simulink model "PID"  (R2023a)
settings: Solver=FixedStepAuto  StartTime=0.0  StopTime=inf  FixedStep=.01  RelTol=1e-3
undefined symbols (not defined in the file or in its folder): angular, linear
libraries: ros2lib x16

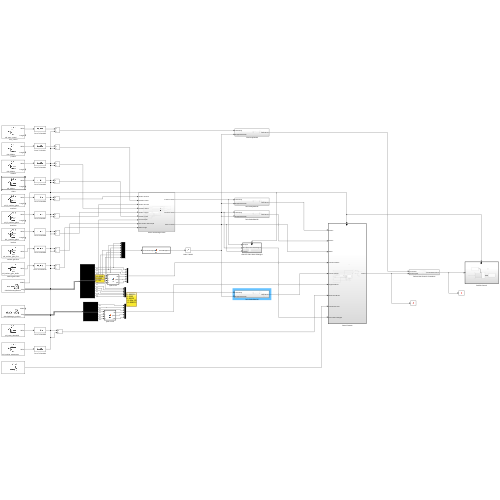
[thumbnail: Simulink's stored preview of the top-level diagram]
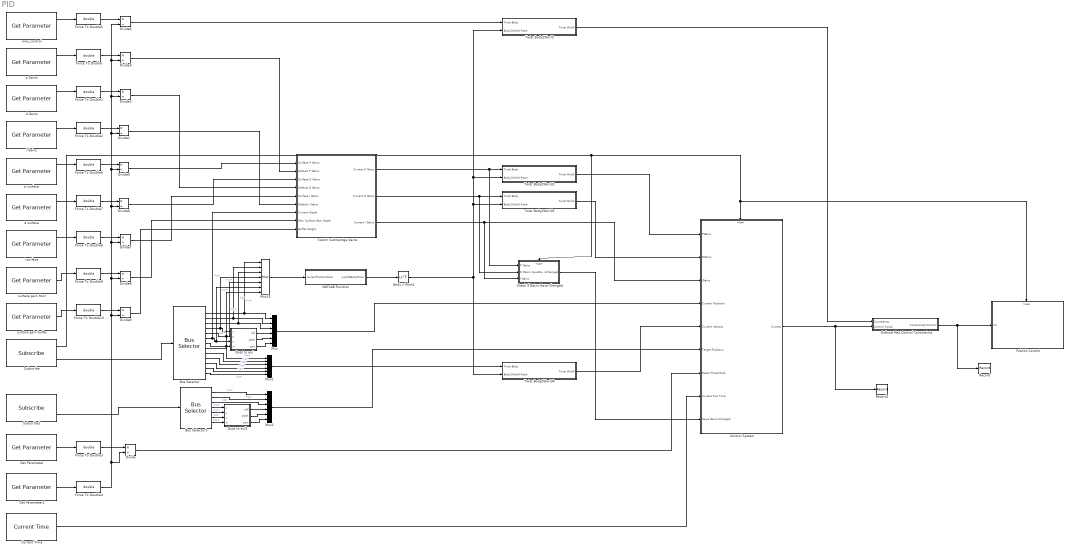
== system PID ==
  Body 2 World : Math  Operator=transpose
  Bus Selector : BusSelector  OutputSignals=pose.pose.position.x,pose.pose.position.y,pose.pose.position.z,pose.pose.orientation.x,pose.pose.orientation.y,pose.pose.orientation.z,pose.pose.orientation.w,twist.twist.linear.x,twist.twist.linear.y,twist.twist.linear.z,twist.twist.angular.x,twist.twist.angular.y,twist.twist.angular.z
  Bus Selector1 : BusSelector  OutputSignals=position.x,position.y,position.z,orientation.x,orientation.y,orientation.z,orientation.w
  Check if Gains Have Changed : Subsystem
  Control System : Subsystem
  Current Time : ros2lib/Current Time  OutputFormat=double  SampleTime=-1  ModelName=PID
  Divide{,1..9} (10 alike) : Product  Inputs=*/
  Enforce Max Control Constraints : Subsystem
  Force To Double{,1..10} (11 alike) : DataTypeConversion  OutDataTypeStr=double  SaturateOnIntegerOverflow=off  RndMeth=Floor
  Get Parameter : ros2lib/Get Parameter  ParameterName=pid_reset_threshold  ParameterType=int64  ParameterMaxArrayLength=16  ParameterInitialValue=100000  SampleTime=-1  ModelName=PID  BlockId=ParamGet_PID_43
  Get Parameter1 : ros2lib/Get Parameter  ParameterName=pid_scaling_parameters  ParameterType=int64  ParameterMaxArrayLength=16  ParameterInitialValue=1000000  SampleTime=-1  ModelName=PID  BlockId=ParamGet_PID_44
  MATLAB Function : MATLAB Function  TreatAsAtomicUnit=on
  Mux : Mux  Inputs=6
  Mux1 : Mux  Inputs=6
  Mux15 : Mux  Inputs=7
  Mux2 : Mux  Inputs=6
  Publish Control : Subsystem
  Quat to eul : MATLAB Function  TreatAsAtomicUnit=on
  Quat to eul1 : MATLAB Function  TreatAsAtomicUnit=on
  Record : Record  FileSettingsInternal="{\"entries\":[{\"content\":{\"excelSettings\":{\"content\":{},\"type\":\"Streamout.ExcelSettings\"}},\"type\":\"Streamout.FileSettingStorage\",\"uuid\":\"\"}],\"packageUris\":[\"http:\\/\\/schema.mathworks.com\\/mf0\\/streamout_blocks\\/R2020a\"],\"version\":\"1.0\"}"  Layout=[1 1]  SignalsInternal="{\"entries\":[{\"content\":{\"signals\":[{\"content\":{\"blockPath\":[],\"dimensions\":[1,6],\"domain\":\"\",\"hasChildren\":true,\"lineColor\":\"#0072bd\",\"port\":1,\"sid\":[\"\"],\"signalID\":55033,\"signalName\":\"Enforce Max Control Constraints\"},\"type\":\"RecordBlkView.Signal\",\"uuid\":\"\"},{\"content\":{\"blockPath\":[],\"channel\":[1,1],\"dimensions\":[1,6],\"domain\":\"\",\"lineColor\":\"#d95319\",\"parentID\":55033,\"port\":1,\"sid\":[\"\"],\"signal ...(+1475 chars)"  VisualizationBindings="{\"sparklinesplugin\":{\"info\":[{\"bindingParametersList\":[],\"subplotID\":1}]}}"
  Record1 : Record  FileSettingsInternal="{\"entries\":[{\"content\":{\"excelSettings\":{\"content\":{},\"type\":\"Streamout.ExcelSettings\"}},\"type\":\"Streamout.FileSettingStorage\",\"uuid\":\"\"}],\"packageUris\":[\"http:\\/\\/schema.mathworks.com\\/mf0\\/streamout_blocks\\/R2020a\"],\"version\":\"1.0\"}"  Layout=[1 1]  SignalsInternal="{\"entries\":[{\"content\":{\"signals\":[{\"content\":{\"blockPath\":[],\"dimensions\":[1,6],\"domain\":\"\",\"hasChildren\":true,\"lineColor\":\"#edb120\",\"port\":1,\"sid\":[\"\"],\"signalID\":55038,\"signalName\":\"Control System\"},\"type\":\"RecordBlkView.Signal\",\"uuid\":\"\"},{\"content\":{\"blockPath\":[],\"channel\":[1,1],\"dimensions\":[1,6],\"domain\":\"\",\"lineColor\":\"#64d413\",\"parentID\":55038,\"plots\":[1],\"port\":1,\"sid\":[\"\"],\"signalID\":5 ...(+1356 chars)"  VisualizationBindings="{\"sparklinesplugin\":{\"info\":[{\"bindingParametersList\":[],\"subplotID\":1}]}}"
  Subscribe : ros2lib/Subscribe  topicSource=Specify your own  topic=/talos/odometry/filtered  messageType=nav_msgs/Odometry  sampleTime=-1  QOSHistory=Keep last  QOSDepth=1  QOSReliability=Reliable  QOSDurability=Volatile
  Subscribe1 : ros2lib/Subscribe  topicSource=Specify your own  topic=/talos/pid/target_position  messageType=geometry_msgs/Pose  sampleTime=-1  QOSHistory=Keep last  QOSDepth=1  QOSReliability=Reliable  QOSDurability=Volatile
  Switch Submerdge Gains : Subsystem
  Twist Body2World : Subsystem
  Twist Body2World1 : Subsystem
  Twist Body2World2 : Subsystem
  Twist Body2World4 : Subsystem
  d Gains : ros2lib/Get Parameter  ParameterName=pid_DGains  ParameterType=int64[]  ParameterMaxArrayLength=6  ParameterInitialValue=[0,0,0,0,0,0]  SampleTime=-1  ModelName=PID  BlockId=ParamGet_PID_47
  d surface : ros2lib/Get Parameter  ParameterName=pid_D_surface_gains  ParameterType=int64[]  ParameterMaxArrayLength=6  ParameterInitialValue=[0,0,0,0,0,0]  SampleTime=-1  ModelName=PID  BlockId=ParamGet_PID_233
  i Gains : ros2lib/Get Parameter  ParameterName=pid_IGains  ParameterType=int64[]  ParameterMaxArrayLength=6  ParameterInitialValue=[0,0,0,0,0,0]  SampleTime=-1  ModelName=PID  BlockId=ParamGet_PID_46
  i surface : ros2lib/Get Parameter  ParameterName=pid_I_surface_gains  ParameterType=int64[]  ParameterMaxArrayLength=6  ParameterInitialValue=[0,0,0,0,0,0]  SampleTime=-1  ModelName=PID  BlockId=ParamGet_PID_234
  max_control : ros2lib/Get Parameter  ParameterName=pid_max_control  ParameterType=int64[]  ParameterMaxArrayLength=6  ParameterInitialValue=[0,0,0,0,0,0]  SampleTime=-1  ModelName=PID  BlockId=ParamGet_PID_123
  p Gains : ros2lib/Get Parameter  ParameterName=pid_PGains  ParameterType=int64[]  ParameterMaxArrayLength=6  ParameterInitialValue=[0,0,0,0,0,0]  SampleTime=-1  ModelName=PID  BlockId=ParamGet_PID_48
  p surface : ros2lib/Get Parameter  ParameterName=pid_P_surface_gains  ParameterType=int64[]  ParameterMaxArrayLength=6  ParameterInitialValue=[0,0,0,0,0,0]  SampleTime=-1  ModelName=PID  BlockId=ParamGet_PID_235
  surface gain buffer : ros2lib/Get Parameter  ParameterName=pid_surface_gain_buffer  ParameterType=int64  ParameterMaxArrayLength=6  ParameterInitialValue=250000  SampleTime=-1  ModelName=PID  BlockId=ParamGet_PID_239
  surface gain floor : ros2lib/Get Parameter  ParameterName=pid_surface_gain_floor  ParameterType=int64  ParameterMaxArrayLength=6  ParameterInitialValue=-750000  SampleTime=-1  ModelName=PID  BlockId=ParamGet_PID_240
  wires:
  Subscribe/2 -> Bus Selector/1
  Bus Selector/4 -> Mux15/4, Quat to eul/1(x)  "<x>"
  Bus Selector/5 -> Mux15/5, Quat to eul/2(y)  "<y>"
  Bus Selector/6 -> Switch Submerdge Gains/7(Current Depth), Mux15/6, Quat to eul/3(z)  "<z>"
  Bus Selector/7 -> Mux15/7, Quat to eul/4(w)  "<w>"
  Quat to eul/3(yaw) -> Mux/6
  Quat to eul/2(pitch) -> Mux/5
  Quat to eul/1(roll) -> Mux/4
  Bus Selector/1 -> Mux15/1, Mux/1  "<x>"
  Bus Selector/2 -> Mux15/2, Mux/2  "<y>"
  Bus Selector/3 -> Mux15/3, Mux/3  "<z>"
  Bus Selector/9 -> Mux1/2  "<y>"
  Bus Selector/8 -> Mux1/1  "<x>"
  Bus Selector/10 -> Mux1/3  "<z>"
  Bus Selector/11 -> Mux1/4  "<x>"
  Bus Selector/12 -> Mux1/5  "<y>"
  Bus Selector/13 -> Mux1/6  "<z>"
  Mux/1 -> Control System/4(Current Positions)
  Subscribe1/2 -> Bus Selector1/1
  Quat to eul1/1(roll) -> Mux2/4
  Quat to eul1/3(yaw) -> Mux2/6
  Quat to eul1/2(pitch) -> Mux2/5
  Get Parameter/1 -> Force To Double3/1
  Get Parameter1/1 -> Force To Double4/1
  Divide/1 -> Control System/7(Reset Threshhold)
  i Gains/1 -> Force To Double2/1
  d Gains/1 -> Force To Double1/1
  p Gains/1 -> Force To Double/1
  Force To Double3/1 -> Divide/1
  Mux2/1 -> Control System/6(Target Positions)
  Bus Selector1/1 -> Mux2/1  "<x>"
  Bus Selector1/2 -> Mux2/2  "<y>"
  Bus Selector1/4 -> Quat to eul1/1(x)  "<x>"
  Bus Selector1/5 -> Quat to eul1/2(y)  "<y>"
  Bus Selector1/6 -> Quat to eul1/3(z)  "<z>"
  Bus Selector1/7 -> Quat to eul1/4(w)  "<w>"
  Bus Selector1/3 -> Mux2/3  "<z>"
  Force To Double2/1 -> Divide1/1
  Force To Double1/1 -> Divide2/1
  Force To Double/1 -> Divide3/1
  Subscribe/1 -> Check if Gains Have Changed/Trigger, Publish Control/Trigger, Control System/Trigger
  MATLAB Function/1(world2BodyRotm) -> Body 2 World/1
  Twist Body2World4/1(Twist World) -> Control System/5(Current Velocity)
  Body 2 World/1 -> Twist Body2World4/2(Body2World Rotm), Twist Body2World2/2(Body2World Rotm), Twist Body2World/2(Body2World Rotm), Twist Body2World1/2(Body2World Rotm)
  Mux15/1 -> MATLAB Function/1(currentPositionQuat)
  max_control/1 -> Force To Double5/1
  Force To Double5/1 -> Divide4/1
  Divide4/1 -> Twist Body2World/1(Twist Body)
  Switch Submerdge Gains/3(Current I Gains) -> Check if Gains Have Changed/3(I Gains), Control System/3(IGains)
  Twist Body2World2/1(Twist World) -> Control System/2(DGains)
  Twist Body2World1/1(Twist World) -> Control System/1(PGains)
  Mux1/1 -> Twist Body2World4/1(Twist Body)
  Twist Body2World/1(Twist World) -> Enforce Max Control Constraints/1(Constraints)
  Control System/1(Control) -> Record1/1, Enforce Max Control Constraints/2(Control Inputs)
  Enforce Max Control Constraints/1(Constrained Control) -> Record/1, Publish Control/1(In1)
  Divide3/1 -> Switch Submerdge Gains/2(Default P Gains)
  Divide2/1 -> Switch Submerdge Gains/4(Default D Gains)
  Divide1/1 -> Switch Submerdge Gains/6(Default I Gains)
  d surface/1 -> Force To Double7/1
  p surface/1 -> Force To Double6/1
  i surface/1 -> Force To Double8/1
  Force To Double8/1 -> Divide7/1
  Force To Double7/1 -> Divide6/1
  Force To Double6/1 -> Divide5/1
  Divide5/1 -> Switch Submerdge Gains/1(Surface P Gains)
  Divide6/1 -> Switch Submerdge Gains/3(Surface D Gains)
  Divide7/1 -> Switch Submerdge Gains/5(Surface I Gains)
  surface gain floor/1 -> Force To Double9/1
  surface gain buffer/1 -> Force To Double10/1
  Force To Double10/1 -> Divide9/1
  Force To Double9/1 -> Divide8/1
  Divide8/1 -> Switch Submerdge Gains/8(Max Surface Gain Depth)
  Divide9/1 -> Switch Submerdge Gains/9(Buffer Height)
  Force To Double4/1 -> Divide/2, Divide9/2, Divide8/2, Divide7/2, Divide6/2, Divide5/2, Divide2/2, Divide3/2, Divide4/2, Divide1/2
  Current Time/1 -> Control System/8(Current Ros Time)
  Switch Submerdge Gains/1(Current P Gains) -> Check if Gains Have Changed/1(P Gains), Twist Body2World1/1(Twist Body)
  Switch Submerdge Gains/2(Current D Gains) -> Check if Gains Have Changed/2(D Gains), Twist Body2World2/1(Twist Body)
  Check if Gains Have Changed/1(haveGainsChanged) -> Control System/9(Have Gains Changed)

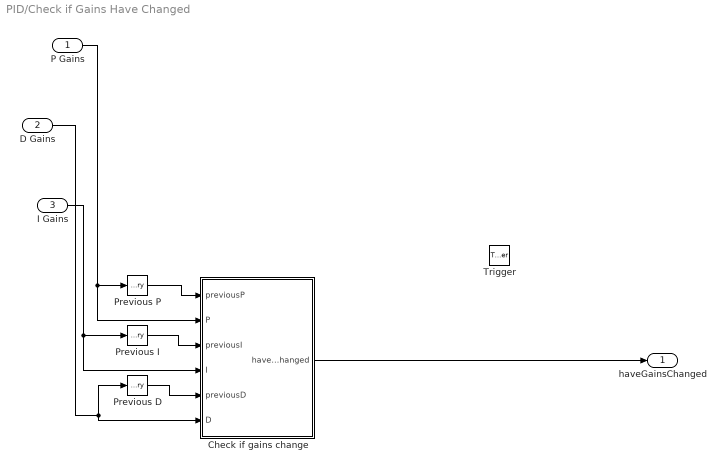
== system PID/Check if Gains Have Changed ==
  P Gains : Inport
  D Gains : Inport  Port=2
  I Gains : Inport  Port=3
  Trigger : TriggerPort  VariantControl=(inherit)  PortDimensions=1
  Check if gains change : MATLAB Function  TreatAsAtomicUnit=on
  Previous D : Memory  InheritSampleTime=on
  Previous I : Memory  InheritSampleTime=on
  Previous P : Memory  InheritSampleTime=on
  haveGainsChanged : Outport
  wires:
  I Gains/1 -> Check if gains change/4(I), Previous I/1
  Previous I/1 -> Check if gains change/3(previousI)
  Previous P/1 -> Check if gains change/1(previousP)
  P Gains/1 -> Check if gains change/2(P), Previous P/1
  Previous D/1 -> Check if gains change/5(previousD)
  D Gains/1 -> Previous D/1, Check if gains change/6(D)
  Check if gains change/1(haveGainsChanged) -> haveGainsChanged/1

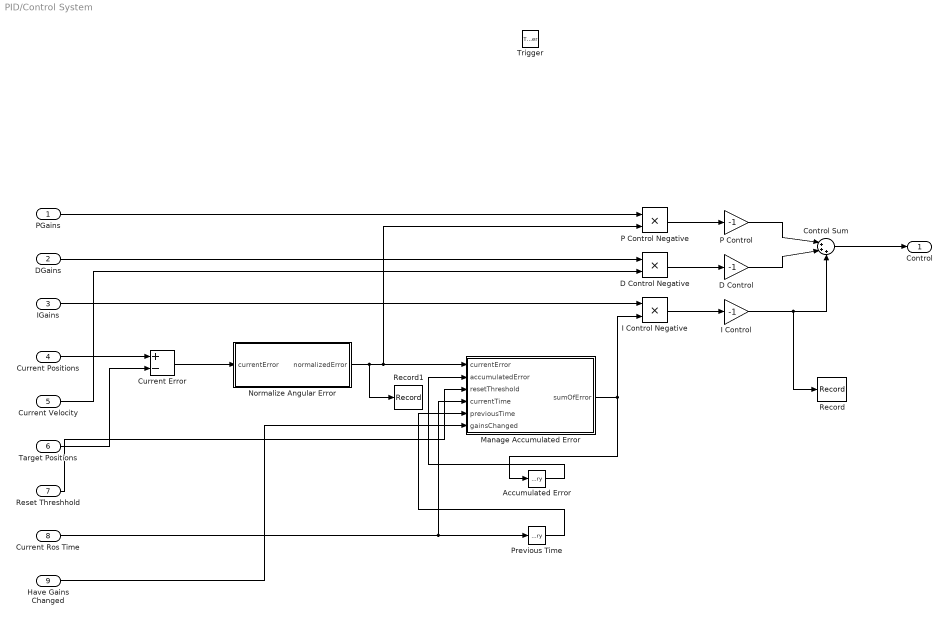
== system PID/Control System ==
  PGains : Inport
  DGains : Inport  Port=2
  IGains : Inport  Port=3
  Current Positions : Inport  Port=4
  Current Velocity : Inport  Port=5
  Target Positions : Inport  Port=6
  Reset Threshhold : Inport  Port=7
  Current Ros Time : Inport  Port=8
  Have Gains Changed : Inport  Port=9
  Trigger : TriggerPort  VariantControl=(inherit)  PortDimensions=1
  Accumulated Error : Memory  InheritSampleTime=on
  Control Sum : Sum  Inputs=|+++
  Current Error : Sum  Inputs=+-
  D Control : Gain  Gain=-1
  D Control Negative : Product
  I Control : Gain  Gain=-1
  I Control Negative : Product
  Manage Accumulated Error : MATLAB Function  TreatAsAtomicUnit=on
  Normalize Angular Error : MATLAB Function  TreatAsAtomicUnit=on
  P Control : Gain  Gain=-1
  P Control Negative : Product
  Previous Time : Memory  InitialCondition=-1  InheritSampleTime=on
  Record : Record  FileSettingsInternal="{\"entries\":[{\"content\":{\"excelSettings\":{\"content\":{},\"type\":\"Streamout.ExcelSettings\"}},\"type\":\"Streamout.FileSettingStorage\",\"uuid\":\"\"}],\"packageUris\":[\"http:\\/\\/schema.mathworks.com\\/mf0\\/streamout_blocks\\/R2020a\"],\"version\":\"1.0\"}"  Layout=[1 1]  SignalsInternal="{\"entries\":[{\"content\":{\"signals\":[{\"content\":{\"blockPath\":[],\"dimensions\":[1,6],\"domain\":\"\",\"hasChildren\":true,\"lineColor\":\"#64d413\",\"port\":1,\"sid\":[\"\"],\"signalID\":55023,\"signalName\":\"I Control\"},\"type\":\"RecordBlkView.Signal\",\"uuid\":\"\"},{\"content\":{\"blockPath\":[],\"channel\":[1,1],\"dimensions\":[1,6],\"domain\":\"\",\"lineColor\":\"#7e2f8e\",\"parentID\":55023,\"port\":1,\"sid\":[\"\"],\"signalID\":55024,\"signalName\" ...(+1297 chars)"  VisualizationBindings="{\"sparklinesplugin\":{\"info\":[{\"bindingParametersList\":[],\"subplotID\":1}]}}"
  Record1 : Record  FileSettingsInternal="{\"entries\":[{\"content\":{\"excelSettings\":{\"content\":{},\"type\":\"Streamout.ExcelSettings\"}},\"type\":\"Streamout.FileSettingStorage\",\"uuid\":\"\"}],\"packageUris\":[\"http:\\/\\/schema.mathworks.com\\/mf0\\/streamout_blocks\\/R2020a\"],\"version\":\"1.0\"}"  Layout=[1 1]  SignalsInternal="{\"entries\":[{\"content\":{\"signals\":[{\"content\":{\"blockPath\":[],\"dimensions\":[1,6],\"domain\":\"\",\"hasChildren\":true,\"lineColor\":\"#fe330a\",\"port\":1,\"sid\":[\"\"],\"signalID\":55028,\"signalName\":\"Normalize Angular Error\"},\"type\":\"RecordBlkView.Signal\",\"uuid\":\"\"},{\"content\":{\"blockPath\":[],\"channel\":[1,1],\"dimensions\":[1,6],\"domain\":\"\",\"lineColor\":\"#edb120\",\"parentID\":55028,\"port\":1,\"sid\":[\"\"],\"signalID\":5502 ...(+1419 chars)"  VisualizationBindings="{\"sparklinesplugin\":{\"info\":[{\"bindingParametersList\":[],\"subplotID\":1}]}}"
  Control : Outport
  wires:
  Reset Threshhold/1 -> Manage Accumulated Error/3(resetThreshold)
  Current Positions/1 -> Current Error/1
  I Control/1 -> Record/1, Control Sum/3
  Current Velocity/1 -> D Control Negative/2
  P Control/1 -> Control Sum/1
  D Control Negative/1 -> D Control/1
  P Control Negative/1 -> P Control/1
  Accumulated Error/1 -> Manage Accumulated Error/2(accumulatedError)
  D Control/1 -> Control Sum/2
  Manage Accumulated Error/1(sumOfError) -> I Control Negative/2, Accumulated Error/1
  I Control Negative/1 -> I Control/1
  Control Sum/1 -> Control/1
  Target Positions/1 -> Current Error/2
  Current Error/1 -> Normalize Angular Error/1(currentError)
  Normalize Angular Error/1(normalizedError) -> Record1/1, P Control Negative/2, Manage Accumulated Error/1(currentError)
  Previous Time/1 -> Manage Accumulated Error/5(previousTime)
  Current Ros Time/1 -> Manage Accumulated Error/4(currentTime), Previous Time/1
  IGains/1 -> I Control Negative/1
  PGains/1 -> P Control Negative/1
  DGains/1 -> D Control Negative/1
  Have Gains Changed/1 -> Manage Accumulated Error/6(gainsChanged)

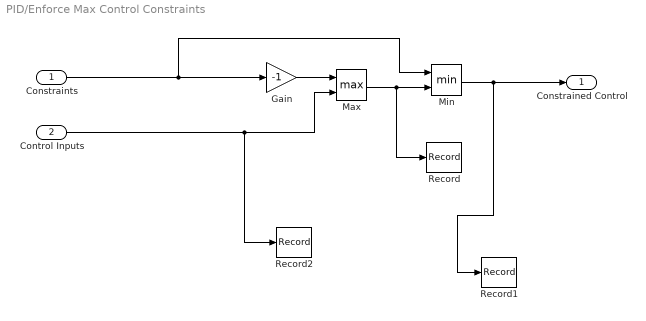
== system PID/Enforce Max Control Constraints ==
  Constraints : Inport
  Control Inputs : Inport  Port=2
  Gain : Gain  Gain=-1
  Max : MinMax  Function=max  Inputs=2
  Min : MinMax  Inputs=2
  Record : Record  FileSettingsInternal="{\"entries\":[{\"content\":{\"excelSettings\":{\"content\":{},\"type\":\"Streamout.ExcelSettings\"}},\"type\":\"Streamout.FileSettingStorage\",\"uuid\":\"\"}],\"packageUris\":[\"http:\\/\\/schema.mathworks.com\\/mf0\\/streamout_blocks\\/R2020a\"],\"version\":\"1.0\"}"  Layout=[1 1]  SignalsInternal="{\"entries\":[{\"content\":{\"signals\":[{\"content\":{\"blockPath\":[],\"dimensions\":[1,6],\"domain\":\"\",\"hasChildren\":true,\"lineColor\":\"#77ac30\",\"port\":1,\"sid\":[\"\"],\"signalID\":55043,\"signalName\":\"Max\"},\"type\":\"RecordBlkView.Signal\",\"uuid\":\"\"},{\"content\":{\"blockPath\":[],\"channel\":[1,1],\"dimensions\":[1,6],\"domain\":\"\",\"lineColor\":\"#0072bd\",\"parentID\":55043,\"port\":1,\"sid\":[\"\"],\"signalID\":55044,\"signalName\":\"Max\" ...(+1255 chars)"  VisualizationBindings="{\"sparklinesplugin\":{\"info\":[{\"bindingParametersList\":[],\"subplotID\":1}]}}"
  Record1 : Record  FileSettingsInternal="{\"entries\":[{\"content\":{\"excelSettings\":{\"content\":{},\"type\":\"Streamout.ExcelSettings\"}},\"type\":\"Streamout.FileSettingStorage\",\"uuid\":\"\"}],\"packageUris\":[\"http:\\/\\/schema.mathworks.com\\/mf0\\/streamout_blocks\\/R2020a\"],\"version\":\"1.0\"}"  Layout=[1 1]  SignalsInternal="{\"entries\":[{\"content\":{\"signals\":[{\"content\":{\"blockPath\":[],\"dimensions\":[1,6],\"domain\":\"\",\"hasChildren\":true,\"lineColor\":\"#a2142f\",\"port\":1,\"sid\":[\"\"],\"signalID\":55048,\"signalName\":\"Min\"},\"type\":\"RecordBlkView.Signal\",\"uuid\":\"\"},{\"content\":{\"blockPath\":[],\"channel\":[1,1],\"dimensions\":[1,6],\"domain\":\"\",\"lineColor\":\"#b746ff\",\"parentID\":55048,\"port\":1,\"sid\":[\"\"],\"signalID\":55049,\"signalName\":\"Min\" ...(+188 chars)"  VisualizationBindings="{\"sparklinesplugin\":{\"info\":[{\"bindingParametersList\":[],\"subplotID\":1}]}}"
  Record2 : Record  FileSettingsInternal="{\"entries\":[{\"content\":{\"excelSettings\":{\"content\":{},\"type\":\"Streamout.ExcelSettings\"}},\"type\":\"Streamout.FileSettingStorage\",\"uuid\":\"\"}],\"packageUris\":[\"http:\\/\\/schema.mathworks.com\\/mf0\\/streamout_blocks\\/R2020a\"],\"version\":\"1.0\"}"  Layout=[1 1]  SignalsInternal="{\"entries\":[{\"content\":{\"signals\":[{\"content\":{\"blockPath\":[],\"dimensions\":[1,6],\"domain\":\"\",\"hasChildren\":true,\"lineColor\":\"#ff6929\",\"port\":1,\"sid\":[\"\"],\"signalID\":55053,\"signalName\":\"Control Inputs\"},\"type\":\"RecordBlkView.Signal\",\"uuid\":\"\"},{\"content\":{\"blockPath\":[],\"channel\":[1,1],\"dimensions\":[1,6],\"domain\":\"\",\"lineColor\":\"#77ac30\",\"parentID\":55053,\"port\":1,\"sid\":[\"\"],\"signalID\":55054,\"signal ...(+1332 chars)"  VisualizationBindings="{\"sparklinesplugin\":{\"info\":[{\"bindingParametersList\":[],\"subplotID\":1}]}}"
  Constrained Control : Outport
  wires:
  Gain/1 -> Max/1
  Min/1 -> Record1/1, Constrained Control/1
  Control Inputs/1 -> Record2/1, Max/2
  Max/1 -> Record/1, Min/2
  Constraints/1 -> Min/1, Gain/1

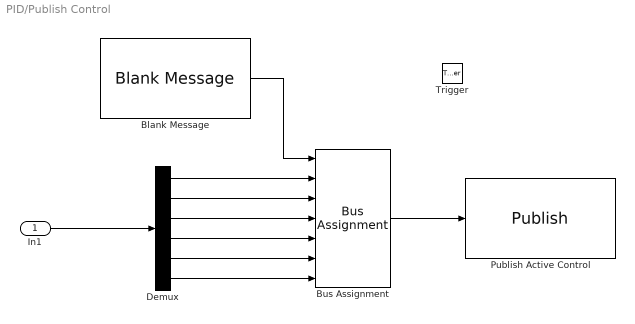
== system PID/Publish Control ==
  In1 : Inport
  Trigger : TriggerPort  VariantControl=(inherit)  PortDimensions=1
  Blank Message : ros2lib/Blank Message  messageClass=Message  entityType=geometry_msgs/Twist  messageType=geometry_msgs/Twist  SampleTime=inf
  Bus Assignment : BusAssignment  AssignedSignals=linear.x,linear.y,linear.z,angular.x,angular.y,angular.z
  Demux : Demux  Outputs=6
  Publish Active Control : ros2lib/Publish  topicSource=Specify your own  topic=/talos/controller/active_body_force  messageType=geometry_msgs/Twist  QOSHistory=Keep last  QOSDepth=1  QOSReliability=Reliable  QOSDurability=Volatile
  wires:
  Blank Message/1 -> Bus Assignment/1
  Demux/1 -> Bus Assignment/2
  Demux/3 -> Bus Assignment/4
  Demux/4 -> Bus Assignment/5
  Demux/5 -> Bus Assignment/6
  Demux/6 -> Bus Assignment/7
  Bus Assignment/1 -> Publish Active Control/1
  In1/1 -> Demux/1
  Demux/2 -> Bus Assignment/3

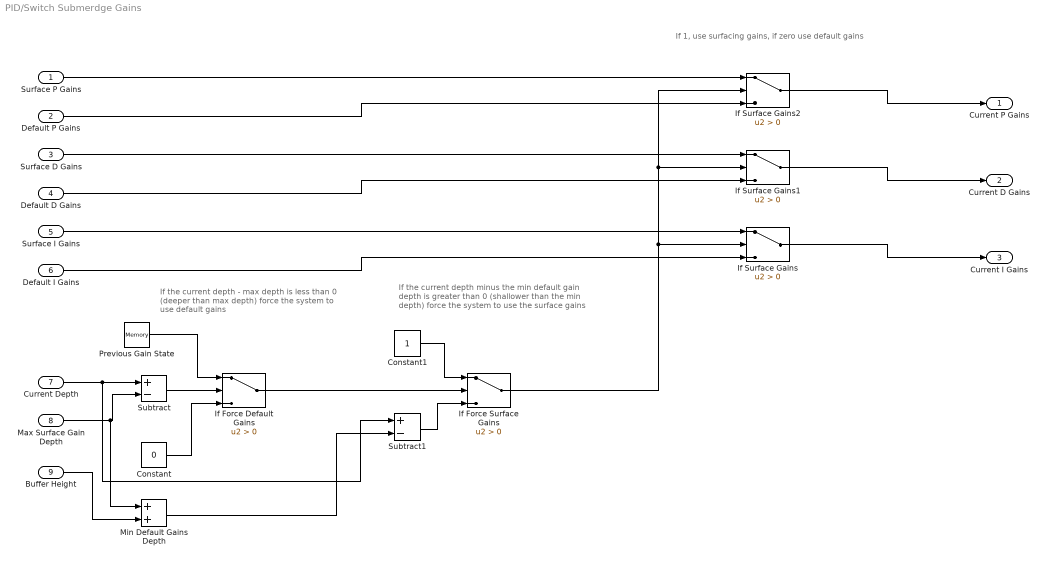
== system PID/Switch Submerdge Gains ==
  note: If the current depth minus the min default gain depth is greater than 0 (shallower than the min depth) force the system to use the surface gains
  note: If the current depth - max depth is less than 0 (deeper than max depth) force the system to use default gains
  note: If 1, use surfacing gains, if zero use default gains
  Surface P Gains : Inport
  Default P Gains : Inport  Port=2
  Surface D Gains : Inport  Port=3
  Default D Gains : Inport  Port=4
  Surface I Gains : Inport  Port=5
  Default I Gains : Inport  Port=6
  Current Depth : Inport  Port=7
  Max Surface Gain Depth : Inport  Port=8
  Buffer Height : Inport  Port=9
  Constant : Constant  Value=0
  Constant1 : Constant
  If Force Default Gains : Switch  Criteria=u2 > Threshold  SaturateOnIntegerOverflow=off  InputSameDT=off
  If Force Surface Gains : Switch  Criteria=u2 > Threshold  SaturateOnIntegerOverflow=off  InputSameDT=off
  If Surface Gains : Switch  Criteria=u2 > Threshold  SaturateOnIntegerOverflow=off  InputSameDT=off
  If Surface Gains1 : Switch  Criteria=u2 > Threshold  SaturateOnIntegerOverflow=off  InputSameDT=off
  If Surface Gains2 : Switch  Criteria=u2 > Threshold  SaturateOnIntegerOverflow=off  InputSameDT=off
  Min Default Gains Depth : Sum
  Previous Gain State : Memory
  Subtract : Sum  Inputs=+-
  Subtract1 : Sum  Inputs=+-
  Current P Gains : Outport
  Current D Gains : Outport  Port=2
  Current I Gains : Outport  Port=3
  wires:
  If Surface Gains1/1 -> Current D Gains/1
  Surface D Gains/1 -> If Surface Gains1/1
  Max Surface Gain Depth/1 -> Min Default Gains Depth/1, Subtract/2
  Surface I Gains/1 -> If Surface Gains/1
  Default I Gains/1 -> If Surface Gains/3
  Surface P Gains/1 -> If Surface Gains2/1
  Current Depth/1 -> Subtract1/1, Subtract/1
  Default D Gains/1 -> If Surface Gains1/3
  Default P Gains/1 -> If Surface Gains2/3
  If Surface Gains/1 -> Current I Gains/1
  If Surface Gains2/1 -> Current P Gains/1
  Subtract/1 -> If Force Default Gains/2
  Constant/1 -> If Force Default Gains/3
  Previous Gain State/1 -> If Force Default Gains/1
  Buffer Height/1 -> Min Default Gains Depth/2
  Min Default Gains Depth/1 -> Subtract1/2
  Subtract1/1 -> If Force Surface Gains/3
  Constant1/1 -> If Force Surface Gains/1
  If Force Default Gains/1 -> If Force Surface Gains/2
  If Force Surface Gains/1 -> If Surface Gains2/2, If Surface Gains1/2, If Surface Gains/2

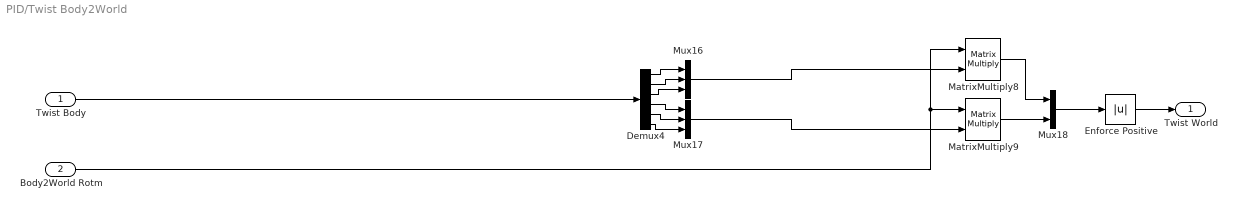
== system PID/Twist Body2World ==
  Twist Body : Inport
  Body2World Rotm : Inport  Port=2
  Demux4 : Demux  Outputs=6
  Enforce Positive : Abs  SaturateOnIntegerOverflow=off
  MatrixMultiply8 : Product  Multiplication=Matrix(*)
  MatrixMultiply9 : Product  Multiplication=Matrix(*)
  Mux16 : Mux  Inputs=3
  Mux17 : Mux  Inputs=3
  Mux18 : Mux  Inputs=2
  Twist World : Outport
  wires:
  Mux17/1 -> MatrixMultiply9/2
  Demux4/2 -> Mux16/2
  Demux4/4 -> Mux17/1
  Mux16/1 -> MatrixMultiply8/2
  Demux4/6 -> Mux17/3
  Demux4/1 -> Mux16/1
  Demux4/5 -> Mux17/2
  MatrixMultiply9/1 -> Mux18/2
  Twist Body/1 -> Demux4/1
  Demux4/3 -> Mux16/3
  Body2World Rotm/1 -> MatrixMultiply8/1, MatrixMultiply9/1
  MatrixMultiply8/1 -> Mux18/1
  Mux18/1 -> Enforce Positive/1
  Enforce Positive/1 -> Twist World/1

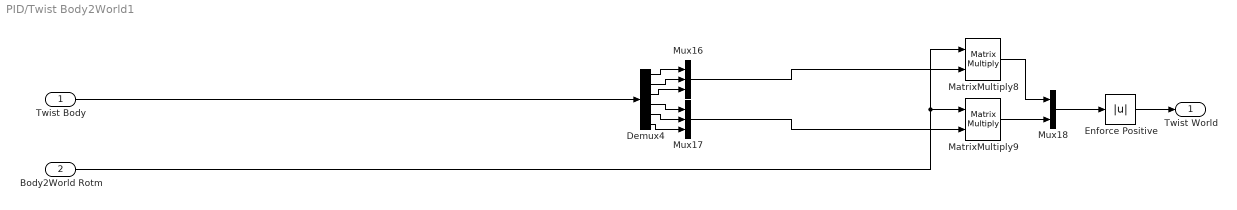
== system PID/Twist Body2World1 ==
  Twist Body : Inport
  Body2World Rotm : Inport  Port=2
  Demux4 : Demux  Outputs=6
  Enforce Positive : Abs  SaturateOnIntegerOverflow=off
  MatrixMultiply8 : Product  Multiplication=Matrix(*)
  MatrixMultiply9 : Product  Multiplication=Matrix(*)
  Mux16 : Mux  Inputs=3
  Mux17 : Mux  Inputs=3
  Mux18 : Mux  Inputs=2
  Twist World : Outport
  wires:
  Mux17/1 -> MatrixMultiply9/2
  Demux4/2 -> Mux16/2
  Demux4/4 -> Mux17/1
  Mux16/1 -> MatrixMultiply8/2
  Demux4/6 -> Mux17/3
  Demux4/1 -> Mux16/1
  Demux4/5 -> Mux17/2
  MatrixMultiply9/1 -> Mux18/2
  Twist Body/1 -> Demux4/1
  Demux4/3 -> Mux16/3
  Body2World Rotm/1 -> MatrixMultiply8/1, MatrixMultiply9/1
  MatrixMultiply8/1 -> Mux18/1
  Mux18/1 -> Enforce Positive/1
  Enforce Positive/1 -> Twist World/1

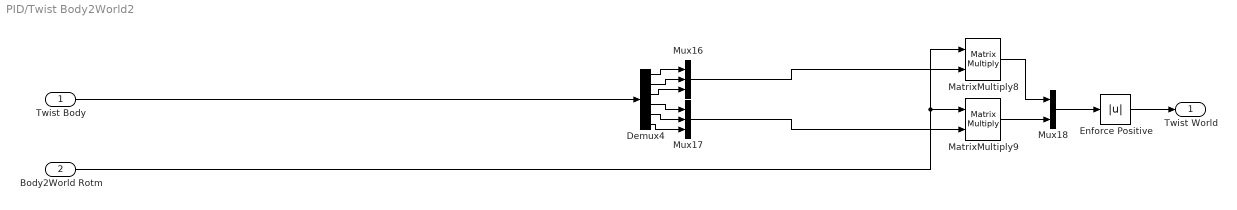
== system PID/Twist Body2World2 ==
  Twist Body : Inport
  Body2World Rotm : Inport  Port=2
  Demux4 : Demux  Outputs=6
  Enforce Positive : Abs  SaturateOnIntegerOverflow=off
  MatrixMultiply8 : Product  Multiplication=Matrix(*)
  MatrixMultiply9 : Product  Multiplication=Matrix(*)
  Mux16 : Mux  Inputs=3
  Mux17 : Mux  Inputs=3
  Mux18 : Mux  Inputs=2
  Twist World : Outport
  wires:
  Mux17/1 -> MatrixMultiply9/2
  Demux4/2 -> Mux16/2
  Demux4/4 -> Mux17/1
  Mux16/1 -> MatrixMultiply8/2
  Demux4/6 -> Mux17/3
  Demux4/1 -> Mux16/1
  Demux4/5 -> Mux17/2
  MatrixMultiply9/1 -> Mux18/2
  Twist Body/1 -> Demux4/1
  Demux4/3 -> Mux16/3
  Body2World Rotm/1 -> MatrixMultiply8/1, MatrixMultiply9/1
  MatrixMultiply8/1 -> Mux18/1
  Mux18/1 -> Enforce Positive/1
  Enforce Positive/1 -> Twist World/1

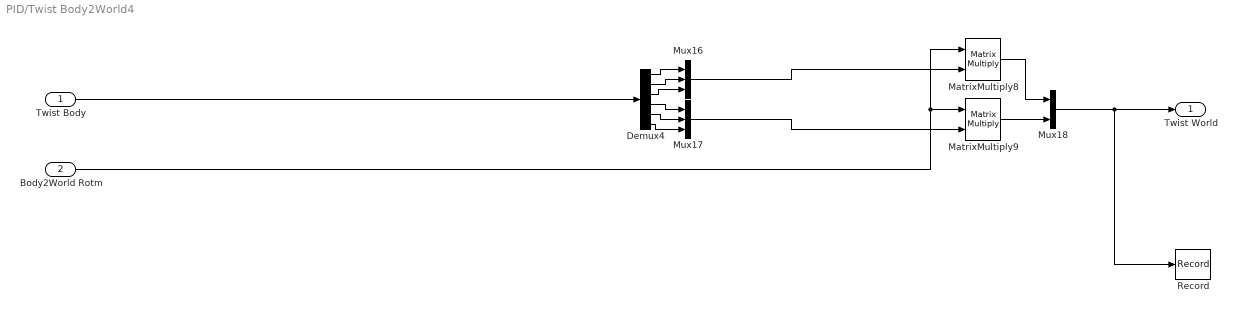
== system PID/Twist Body2World4 ==
  Twist Body : Inport
  Body2World Rotm : Inport  Port=2
  Demux4 : Demux  Outputs=6
  MatrixMultiply8 : Product  Multiplication=Matrix(*)
  MatrixMultiply9 : Product  Multiplication=Matrix(*)
  Mux16 : Mux  Inputs=3
  Mux17 : Mux  Inputs=3
  Mux18 : Mux  Inputs=2
  Record : Record  FileSettingsInternal="{\"entries\":[{\"content\":{\"excelSettings\":{\"content\":{},\"type\":\"Streamout.ExcelSettings\"}},\"type\":\"Streamout.FileSettingStorage\",\"uuid\":\"\"}],\"packageUris\":[\"http:\\/\\/schema.mathworks.com\\/mf0\\/streamout_blocks\\/R2020a\"],\"version\":\"1.0\"}"  Layout=[1 1]  SignalsInternal="{\"entries\":[{\"content\":{\"signals\":[{\"content\":{\"blockPath\":[],\"dimensions\":[6],\"domain\":\"\",\"hasChildren\":true,\"lineColor\":\"#64d413\",\"port\":1,\"sid\":[\"\"],\"signalID\":55058,\"signalName\":\"Mux18\"},\"type\":\"RecordBlkView.Signal\",\"uuid\":\"\"},{\"content\":{\"blockPath\":[],\"channel\":[1],\"dimensions\":[6],\"domain\":\"\",\"lineColor\":\"#ff13a6\",\"parentID\":55058,\"plots\":[1],\"port\":1,\"sid\":[\"\"],\"signalID\":55059,\"signalNam ...(+1267 chars)"  VisualizationBindings="{\"sparklinesplugin\":{\"info\":[{\"bindingParametersList\":[],\"subplotID\":1}]}}"
  Twist World : Outport
  wires:
  Mux17/1 -> MatrixMultiply9/2
  Demux4/2 -> Mux16/2
  Demux4/4 -> Mux17/1
  Mux16/1 -> MatrixMultiply8/2
  Demux4/6 -> Mux17/3
  Demux4/1 -> Mux16/1
  Demux4/5 -> Mux17/2
  MatrixMultiply9/1 -> Mux18/2
  Twist Body/1 -> Demux4/1
  Demux4/3 -> Mux16/3
  Body2World Rotm/1 -> MatrixMultiply8/1, MatrixMultiply9/1
  MatrixMultiply8/1 -> Mux18/1
  Mux18/1 -> Record/1, Twist World/1

== matlab function PID/Quat to eul ==
function [roll, pitch, yaw] = fcn(x,y,z,w)

%convert the quaternion to euler
euler = quat2eul([w,x,y,z]);

roll = euler(3);
pitch = euler(2);
yaw = euler(1);

== matlab function PID/Control System/Manage Accumulated Error ==
function sumOfError = fcn(currentError, accumulatedError, resetThreshold, currentTime, previousTime, gainsChanged)

deltaTime = 0;
if(previousTime <= 0)
    sumOfError = zeros(1,6);
    return 
else
    deltaTime = currentTime - previousTime;
end

sum = zeros(1,6);

%if gains get reset, reset accumulator
if(gainsChanged)
   sumOfError = zeros(1,6);

   disp(gainsChanged)

   return
end

%check each degree of freedom
for i = 1:6
    sum(i) = (currentError(i)) * deltaTime + accumulatedError(i);

    if(currentError(i) > resetThreshold)
        sum(i) = 0;
    end

    %reset if nan
    if(isnan(currentError(i)))
        sum(i) = 0;
    end

end

sumOfError = sum;

== matlab function PID/Control System/Normalize Angular Error ==
function normalizedError = fcn(currentError)

normalized = zeros(1,6);

normalized(1) = currentError(1);
normalized(2) = currentError(2);
normalized(3) = currentError(3);

%each angular degree of freedom
for i=4:6
    %normalize all error to between postive and negative 180
    normalized(i) = mod(currentError(i) + pi, 2 * pi) - pi;
end

normalizedError = normalized;

== matlab function PID/Quat to eul1 ==
function [roll, pitch, yaw] = fcn(x,y,z,w)

%convert the quaternion to euler
euler = quat2eul([w,x,y,z]);

roll = euler(3);
pitch = euler(2);
yaw = euler(1);

if(isnan(roll))
   roll = 0;
   pitch = 0;
   yaw = 0;
end

== matlab function PID/MATLAB Function ==
function world2BodyRotm = fcn(currentPositionQuat)


world2BodyRotm = quat2rotm([currentPositionQuat(7), currentPositionQuat(4), currentPositionQuat(5), currentPositionQuat(6)]);

== matlab function PID/Check if Gains Have Changed/Check if gains change ==
function haveGainsChanged  = fcn(previousP, P, previousI, I, previousD, D)


%check if P gains have changed
if(~isequal(P, previousP))
    haveGainsChanged = true;
    return
end


%check if  I gains have changed
if(~isequal(I, previousI))
    haveGainsChanged = true;
    return
end


%check if  D gains have changed
if(~isequal(D, previousD))
    haveGainsChanged = true;
    return
end

haveGainsChanged = false;
